simulink model "RM3_instf_ctrl_clean"  (R2024b)
settings: Solver=FixedStepAuto  StartTime=0.0  StopTime=1200  FixedStep=0.1  MaxStep=1e-3  RelTol=1e-7
values from neighbouring files (symbols this model uses):
  estimation_method_selection = 2    [RM3_instf_init.m]
  fp = 1/9    (= 0.111111111111)    [PLL_script_MDPI.m]    (also in RM3_instf_init.m)
  pto_damping_values = zeros(size(hydro.w))    [RM3_instf_init.m]    (also in lookup_table_data.mat = [17367795.7359 18541234.6755 40743919.319 43726293.4916 5082)
  pto_stiffness_values = zeros(size(hydro.w))    [RM3_instf_init.m]    (also in lookup_table_data.mat = [0 0 0 0 0 0 0 0 0 0 0 0 ... (260 elements, 1x260)])
undefined symbols (not defined in the file or in its folder): rm3_ss_0p1
libraries: eeSinusoidalMeasurementV2 x1, dspsigops x1
settings Model: Creator=inyongkim  LastModifiedBy=inyongkim

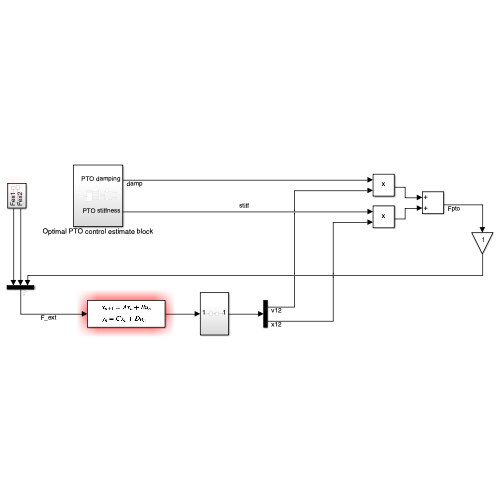
[thumbnail: Simulink's stored preview of the top-level diagram]
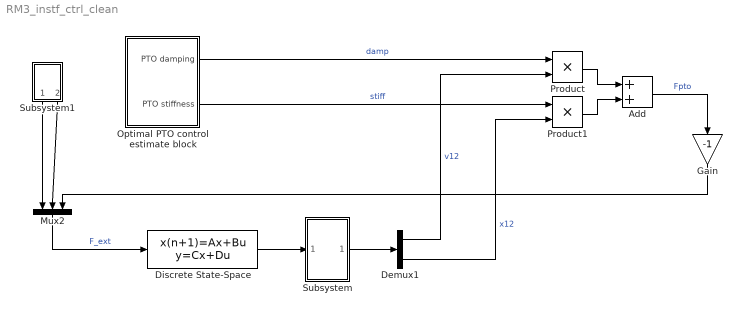
== system RM3_instf_ctrl_clean ==
  Add : Sum
  Demux1 : Demux  Outputs=2
  Discrete State-Space : DiscreteStateSpace  A=rm3_ss_0p1.A  B=rm3_ss_0p1.B  C=rm3_ss_0p1.C  D=rm3_ss_0p1.D  SampleTime=0.1
  Gain : Gain  Gain=-1
  Mux2 : Mux  Inputs=3
  Optimal PTO control estimate block : Subsystem
  Product : Product
  Product1 : Product
  Subsystem : Subsystem
  Subsystem1 : Subsystem
  wires:
  Demux1/2 -> Product1/2  "x12"
  Product/1 -> Add/1
  Product1/1 -> Add/2
  Add/1 -> Gain/1  "Fpto"
  Mux2/1 -> Discrete State-Space/1  "F_ext"
  Optimal PTO control estimate block/1(PTO damping) -> Product/1  "damp"
  Optimal PTO control estimate block/2(PTO stiffness) -> Product1/1  "stiff"
  Gain/1 -> Mux2/3
  Demux1/1 -> Product/2  "v12"
  Discrete State-Space/1 -> Subsystem/1(In1)
  Subsystem/1(Out1) -> Demux1/1
  Subsystem1/1(Fex1) -> Mux2/1
  Subsystem1/2(Fex2) -> Mux2/2

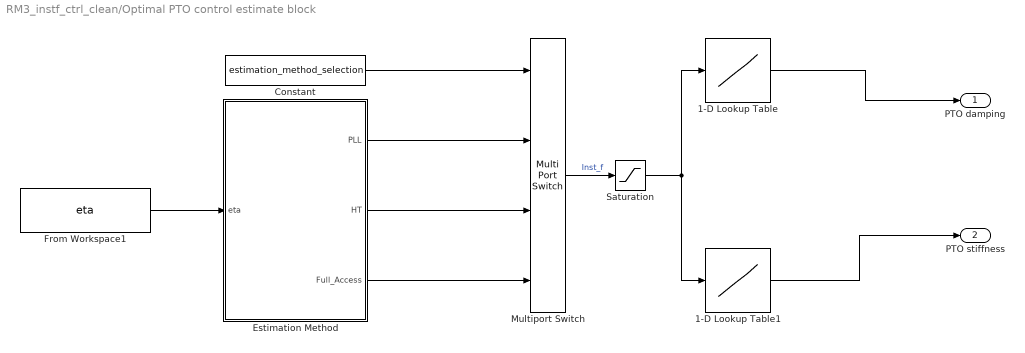
== system RM3_instf_ctrl_clean/Optimal PTO control estimate block ==
  1-D Lookup Table : Lookup_n-D  NumberOfTableDimensions=1  BreakpointsForDimension1=w_ref/2/pi  Table=pto_damping_values  InternalRulePriority=Speed  RndMeth=Simplest
  1-D Lookup Table1 : Lookup_n-D  NumberOfTableDimensions=1  BreakpointsForDimension1=w_ref/2/pi  Table=pto_stiffness_values  InternalRulePriority=Speed  RndMeth=Simplest
  Constant : Constant  Value=estimation_method_selection
  Estimation Method : Subsystem
  From Workspace1 : FromWorkspace  VariableName=eta
  Multiport Switch : MultiPortSwitch  SaturateOnIntegerOverflow=off  InputSameDT=off
  Saturation : Saturate  UpperLimit=fp*1.15  LowerLimit=fp*0.01
  PTO damping : Outport
  PTO stiffness : Outport  Port=2
  wires:
  Multiport Switch/1 -> Saturation/1  "Inst_f"
  1-D Lookup Table/1 -> PTO damping/1
  1-D Lookup Table1/1 -> PTO stiffness/1
  Saturation/1 -> 1-D Lookup Table1/1, 1-D Lookup Table/1
  Constant/1 -> Multiport Switch/1
  From Workspace1/1 -> Estimation Method/1(eta)
  Estimation Method/1(PLL) -> Multiport Switch/2
  Estimation Method/2(HT) -> Multiport Switch/3
  Estimation Method/3(Full_Access) -> Multiport Switch/4

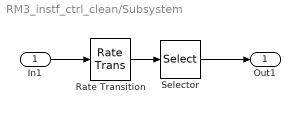
== system RM3_instf_ctrl_clean/Subsystem ==
  In1 : Inport
  Rate Transition : RateTransition  OutPortSampleTime=0
  Selector : Selector  InputPortWidth=6  IndexOptions=Index vector (dialog)  Indices=[5 6]  OutputSizes=1
  Out1 : Outport
  wires:
  In1/1 -> Rate Transition/1
  Selector/1 -> Out1/1
  Rate Transition/1 -> Selector/1

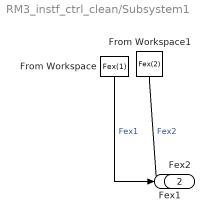
== system RM3_instf_ctrl_clean/Subsystem1 ==
  From Workspace : FromWorkspace  VariableName=Fex(1)
  From Workspace1 : FromWorkspace  VariableName=Fex(2)
  Fex1 : Outport
  Fex2 : Outport  Port=2
  wires:
  From Workspace/1 -> Fex1/1  "Fex1"
  From Workspace1/1 -> Fex2/1  "Fex2"

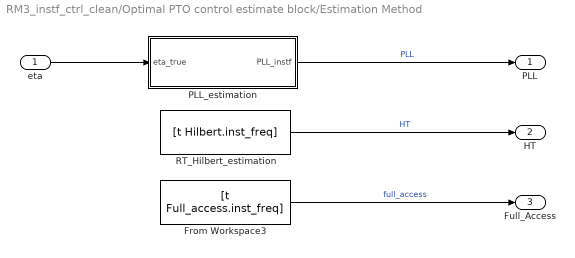
== system RM3_instf_ctrl_clean/Optimal PTO control estimate block/Estimation Method ==
  eta : Inport
  From Workspace3 : FromWorkspace  VariableName=[t Full_access.inst_freq]
  PLL_estimation : Subsystem
  RT_Hilbert_estimation : FromWorkspace  VariableName=[t Hilbert.inst_freq]
  PLL : Outport
  HT : Outport  Port=2
  Full_Access : Outport  Port=3
  wires:
  PLL_estimation/1(PLL_instf) -> PLL/1  "PLL"
  RT_Hilbert_estimation/1 -> HT/1  "HT"
  From Workspace3/1 -> Full_Access/1  "full_access"
  eta/1 -> PLL_estimation/1(eta_true)

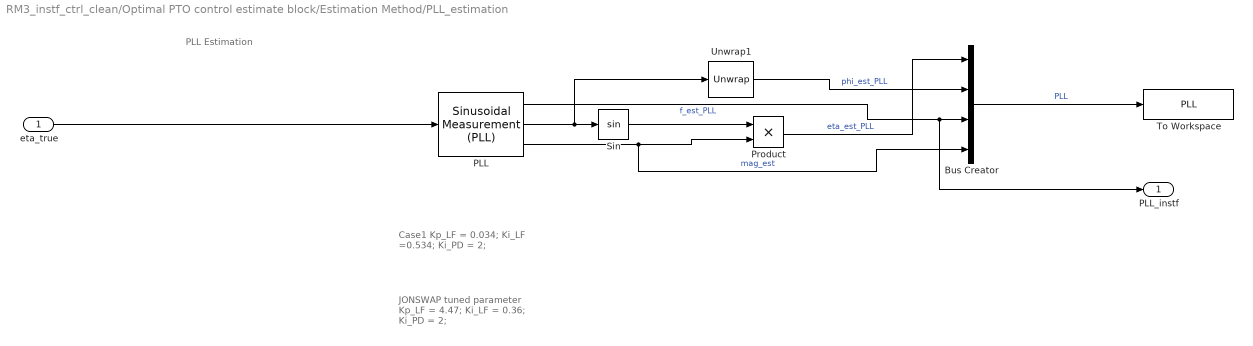
== system RM3_instf_ctrl_clean/Optimal PTO control estimate block/Estimation Method/PLL_estimation ==
  note: JONSWAP tuned parameter
      | Kp_LF = 4.47;
      | Ki_LF = 0.36;
      | Ki_PD = 2;
  note: PLL Estimation
  note: Case1
      | Kp_LF = 0.034;
      | Ki_LF =0.534;
      | Ki_PD = 2;
  eta_true : Inport
  Bus Creator : BusCreator  Inputs=4
  PLL : eeSinusoidalMeasurementV2/Sinusoidal Measurement (PLL)  Ki_PD=2  Kp_LF=Kp_LF  Ki_LF=Ki_LF  F0=wbar/2/pi  Theta0=0  Mag0=1  Ts=-1
      settings: LibrarySourceBlock=|
      | ee_sl_lib/Measurements/Sinusoidal Measurement
      | (PLL)
  Product : Product
  Sin : Trigonometry
  To Workspace : ToWorkspace  VariableName=PLL  SaveFormat=Timeseries  SampleTime=-1
  Unwrap1 : dspsigops/Unwrap  tol=pi  running=off
  PLL_instf : Outport
  wires:
  Unwrap1/1 -> Bus Creator/2  "phi_est_PLL"
  Product/1 -> Bus Creator/1  "eta_est_PLL"
  eta_true/1 -> PLL/1
  PLL/2 -> Unwrap1/1, Sin/1
  Sin/1 -> Product/1
  PLL/1 -> PLL_instf/1, Bus Creator/3  "f_est_PLL"
  Bus Creator/1 -> To Workspace/1  "PLL"
  PLL/3 -> Bus Creator/4, Product/2  "mag_est"
